simulink model "Kalman_gefiltert"  (R2019b)
settings: Solver=VariableStepAuto  StartTime=0.0  StopTime=750  RelTol=1e-3
undefined symbols (not defined in the file or in its folder): Discrete, Time
libraries: ctrlSharedLib x9

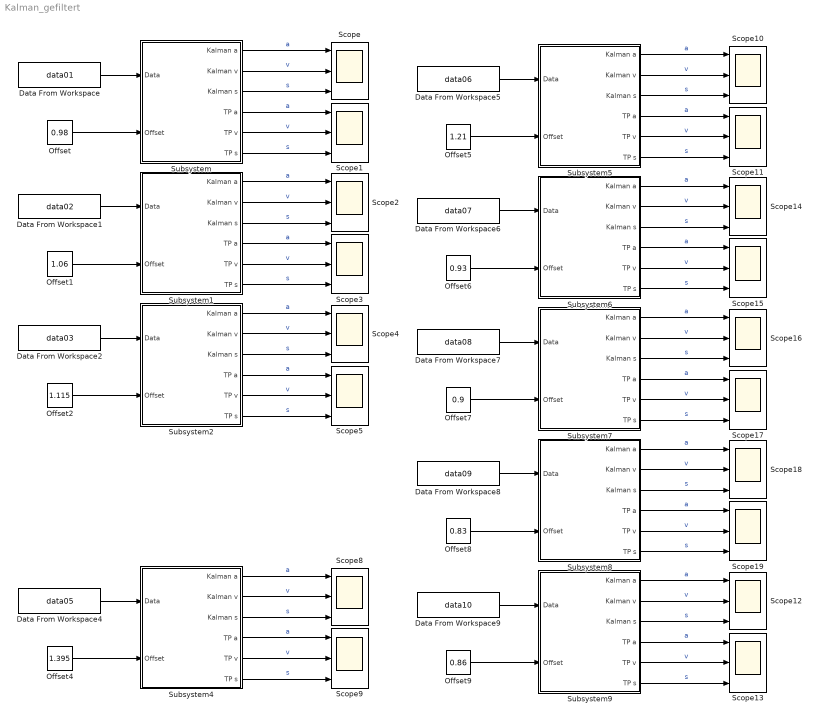
== system Kalman_gefiltert ==
  Data From Workspace : FromWorkspace  VariableName=data01  SampleTime=0
  Data From Workspace1 : FromWorkspace  VariableName=data02  SampleTime=0
  Data From Workspace2 : FromWorkspace  VariableName=data03  SampleTime=0
  Data From Workspace4 : FromWorkspace  VariableName=data05  SampleTime=0
  Data From Workspace5 : FromWorkspace  VariableName=data06  SampleTime=0
  Data From Workspace6 : FromWorkspace  VariableName=data07  SampleTime=0
  Data From Workspace7 : FromWorkspace  VariableName=data08  SampleTime=0
  Data From Workspace8 : FromWorkspace  VariableName=data09  SampleTime=0
  Data From Workspace9 : FromWorkspace  VariableName=data10  SampleTime=0
  Offset : Constant  Value=0.98
  Offset1 : Constant  Value=1.06
  Offset2 : Constant  Value=1.115
  Offset4 : Constant  Value=1.395
  Offset5 : Constant  Value=1.21
  Offset6 : Constant  Value=0.93
  Offset7 : Constant  Value=0.9
  Offset8 : Constant  Value=0.83
  Offset9 : Constant  Value=0.86
  Scope{,1..5,8..19} (18 alike) : Scope  NumInputPorts=3
  Subsystem : Subsystem
  Subsystem1 : Subsystem
  Subsystem2 : Subsystem
  Subsystem4 : Subsystem
  Subsystem5 : Subsystem
  Subsystem6 : Subsystem
  Subsystem7 : Subsystem
  Subsystem8 : Subsystem
  Subsystem9 : Subsystem
  wires:
  Data From Workspace/1 -> Subsystem/1(Data)
  Offset/1 -> Subsystem/2(Offset)
  Subsystem/1(Kalman a) -> Scope/1  "a"
  Subsystem/2(Kalman v) -> Scope/2  "v"
  Subsystem/3(Kalman s) -> Scope/3  "s"
  Subsystem/4(TP a) -> Scope1/1  "a"
  Subsystem/5(TP v) -> Scope1/2  "v"
  Subsystem/6(TP s) -> Scope1/3  "s"
  Subsystem1/6(TP s) -> Scope3/3  "s"
  Subsystem1/5(TP v) -> Scope3/2  "v"
  Subsystem1/3(Kalman s) -> Scope2/3  "s"
  Offset1/1 -> Subsystem1/2(Offset)
  Subsystem1/2(Kalman v) -> Scope2/2  "v"
  Subsystem1/4(TP a) -> Scope3/1  "a"
  Subsystem1/1(Kalman a) -> Scope2/1  "a"
  Data From Workspace2/1 -> Subsystem2/1(Data)
  Subsystem2/6(TP s) -> Scope5/3  "s"
  Subsystem2/5(TP v) -> Scope5/2  "v"
  Subsystem2/3(Kalman s) -> Scope4/3  "s"
  Offset2/1 -> Subsystem2/2(Offset)
  Subsystem2/2(Kalman v) -> Scope4/2  "v"
  Subsystem2/4(TP a) -> Scope5/1  "a"
  Subsystem2/1(Kalman a) -> Scope4/1  "a"
  Subsystem5/2(Kalman v) -> Scope10/2  "v"
  Subsystem5/1(Kalman a) -> Scope10/1  "a"
  Offset5/1 -> Subsystem5/2(Offset)
  Subsystem5/4(TP a) -> Scope11/1  "a"
  Subsystem5/5(TP v) -> Scope11/2  "v"
  Subsystem5/3(Kalman s) -> Scope10/3  "s"
  Data From Workspace5/1 -> Subsystem5/1(Data)
  Subsystem4/1(Kalman a) -> Scope8/1  "a"
  Offset4/1 -> Subsystem4/2(Offset)
  Subsystem4/3(Kalman s) -> Scope8/3  "s"
  Subsystem4/2(Kalman v) -> Scope8/2  "v"
  Subsystem4/5(TP v) -> Scope9/2  "v"
  Data From Workspace4/1 -> Subsystem4/1(Data)
  Subsystem4/4(TP a) -> Scope9/1  "a"
  Subsystem4/6(TP s) -> Scope9/3  "s"
  Subsystem5/6(TP s) -> Scope11/3  "s"
  Subsystem7/1(Kalman a) -> Scope16/1  "a"
  Subsystem9/6(TP s) -> Scope13/3  "s"
  Subsystem8/6(TP s) -> Scope19/3  "s"
  Data From Workspace8/1 -> Subsystem8/1(Data)
  Subsystem8/1(Kalman a) -> Scope18/1  "a"
  Subsystem8/4(TP a) -> Scope19/1  "a"
  Subsystem8/5(TP v) -> Scope19/2  "v"
  Subsystem7/3(Kalman s) -> Scope16/3  "s"
  Offset9/1 -> Subsystem9/2(Offset)
  Subsystem9/4(TP a) -> Scope13/1  "a"
  Data From Workspace9/1 -> Subsystem9/1(Data)
  Subsystem9/3(Kalman s) -> Scope12/3  "s"
  Subsystem8/2(Kalman v) -> Scope18/2  "v"
  Subsystem9/5(TP v) -> Scope13/2  "v"
  Subsystem7/4(TP a) -> Scope17/1  "a"
  Data From Workspace7/1 -> Subsystem7/1(Data)
  Subsystem7/2(Kalman v) -> Scope16/2  "v"
  Subsystem8/3(Kalman s) -> Scope18/3  "s"
  Offset7/1 -> Subsystem7/2(Offset)
  Subsystem7/6(TP s) -> Scope17/3  "s"
  Subsystem6/1(Kalman a) -> Scope14/1  "a"
  Offset6/1 -> Subsystem6/2(Offset)
  Subsystem9/1(Kalman a) -> Scope12/1  "a"
  Offset8/1 -> Subsystem8/2(Offset)
  Subsystem6/4(TP a) -> Scope15/1  "a"
  Subsystem6/5(TP v) -> Scope15/2  "v"
  Subsystem6/2(Kalman v) -> Scope14/2  "v"
  Subsystem7/5(TP v) -> Scope17/2  "v"
  Data From Workspace6/1 -> Subsystem6/1(Data)
  Subsystem6/6(TP s) -> Scope15/3  "s"
  Subsystem6/3(Kalman s) -> Scope14/3  "s"
  Subsystem9/2(Kalman v) -> Scope12/2  "v"
  Data From Workspace1/1 -> Subsystem1/1(Data)

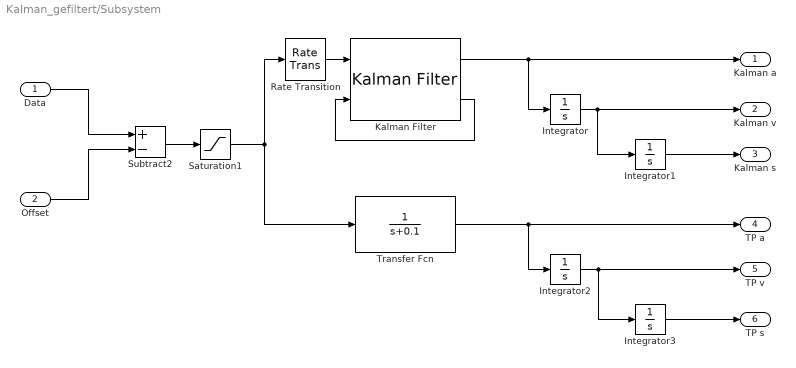
== system Kalman_gefiltert/Subsystem ==
  Data : Inport
  Offset : Inport  Port=2
  Integrator{,1..3} (4 alike) : Integrator
  Kalman Filter : ctrlSharedLib/Kalman Filter  TimeDomain=Discrete-Time  UseCurrentEstimator=on  ModelSource=LTI State-Space Variable  ModelSourceVariable=ss(0.95,1,1,0,1)  A=0.95  B=1  C=1  D=0  NumberOfStates=1  NumberOfInputs=1  NumberOfOutputs=1  InitialEstimateSource=Dialog  X0=0  P0=10  UseK=off  UseGH=off  NumberOfProcessNoiseInputs=1  G=1  TimeInvariantG=on  H=0  TimeInvariantH=on  Q=0.05  TimeInvariantQ=on  R=1  TimeInvariantR=on  N=0  TimeInvariantN=on  AddInputPort=on  AddEnablePort=off  OutputEstimatedY=on  OutputP=off  Ts=-1
  Rate Transition : RateTransition
  Saturation1 : Saturate  UpperLimit=inf  LowerLimit=0
  Subtract2 : Sum  Inputs=+-
  Transfer Fcn : TransferFcn  Denominator=[1 0.1]
  Kalman a : Outport
  Kalman v : Outport  Port=2
  Kalman s : Outport  Port=3
  TP a : Outport  Port=4
  TP v : Outport  Port=5
  TP s : Outport  Port=6
  wires:
  Integrator2/1 -> TP v/1, Integrator3/1
  Integrator3/1 -> TP s/1
  Kalman Filter/2 -> Kalman Filter/2
  Data/1 -> Subtract2/1
  Offset/1 -> Subtract2/2
  Integrator/1 -> Kalman v/1, Integrator1/1
  Transfer Fcn/1 -> TP a/1, Integrator2/1
  Subtract2/1 -> Saturation1/1
  Kalman Filter/1 -> Kalman a/1, Integrator/1
  Integrator1/1 -> Kalman s/1
  Saturation1/1 -> Transfer Fcn/1, Rate Transition/1
  Rate Transition/1 -> Kalman Filter/1

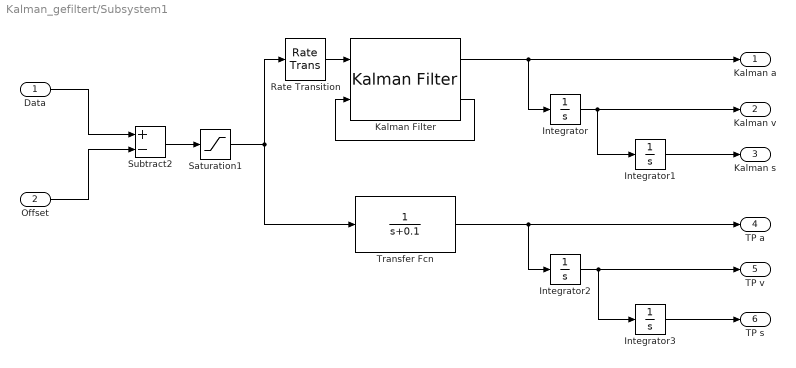
== system Kalman_gefiltert/Subsystem1 ==
  Data : Inport
  Offset : Inport  Port=2
  Integrator{,1..3} (4 alike) : Integrator
  Kalman Filter : ctrlSharedLib/Kalman Filter  TimeDomain=Discrete-Time  UseCurrentEstimator=on  ModelSource=LTI State-Space Variable  ModelSourceVariable=ss(0.95,1,1,0,1)  A=0.95  B=1  C=1  D=0  NumberOfStates=1  NumberOfInputs=1  NumberOfOutputs=1  InitialEstimateSource=Dialog  X0=0  P0=10  UseK=off  UseGH=off  NumberOfProcessNoiseInputs=1  G=1  TimeInvariantG=on  H=0  TimeInvariantH=on  Q=0.05  TimeInvariantQ=on  R=1  TimeInvariantR=on  N=0  TimeInvariantN=on  AddInputPort=on  AddEnablePort=off  OutputEstimatedY=on  OutputP=off  Ts=-1
  Rate Transition : RateTransition
  Saturation1 : Saturate  UpperLimit=inf  LowerLimit=0
  Subtract2 : Sum  Inputs=+-
  Transfer Fcn : TransferFcn  Denominator=[1 0.1]
  Kalman a : Outport
  Kalman v : Outport  Port=2
  Kalman s : Outport  Port=3
  TP a : Outport  Port=4
  TP v : Outport  Port=5
  TP s : Outport  Port=6
  wires:
  Integrator2/1 -> TP v/1, Integrator3/1
  Integrator3/1 -> TP s/1
  Kalman Filter/2 -> Kalman Filter/2
  Data/1 -> Subtract2/1
  Offset/1 -> Subtract2/2
  Integrator/1 -> Kalman v/1, Integrator1/1
  Transfer Fcn/1 -> TP a/1, Integrator2/1
  Subtract2/1 -> Saturation1/1
  Kalman Filter/1 -> Kalman a/1, Integrator/1
  Integrator1/1 -> Kalman s/1
  Saturation1/1 -> Transfer Fcn/1, Rate Transition/1
  Rate Transition/1 -> Kalman Filter/1

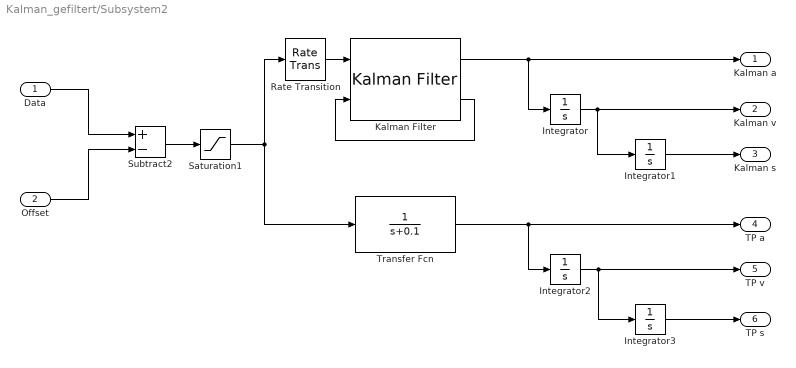
== system Kalman_gefiltert/Subsystem2 ==
  Data : Inport
  Offset : Inport  Port=2
  Integrator{,1..3} (4 alike) : Integrator
  Kalman Filter : ctrlSharedLib/Kalman Filter  TimeDomain=Discrete-Time  UseCurrentEstimator=on  ModelSource=LTI State-Space Variable  ModelSourceVariable=ss(0.95,1,1,0,1)  A=0.95  B=1  C=1  D=0  NumberOfStates=1  NumberOfInputs=1  NumberOfOutputs=1  InitialEstimateSource=Dialog  X0=0  P0=10  UseK=off  UseGH=off  NumberOfProcessNoiseInputs=1  G=1  TimeInvariantG=on  H=0  TimeInvariantH=on  Q=0.05  TimeInvariantQ=on  R=1  TimeInvariantR=on  N=0  TimeInvariantN=on  AddInputPort=on  AddEnablePort=off  OutputEstimatedY=on  OutputP=off  Ts=-1
  Rate Transition : RateTransition
  Saturation1 : Saturate  UpperLimit=inf  LowerLimit=0
  Subtract2 : Sum  Inputs=+-
  Transfer Fcn : TransferFcn  Denominator=[1 0.1]
  Kalman a : Outport
  Kalman v : Outport  Port=2
  Kalman s : Outport  Port=3
  TP a : Outport  Port=4
  TP v : Outport  Port=5
  TP s : Outport  Port=6
  wires:
  Integrator2/1 -> TP v/1, Integrator3/1
  Integrator3/1 -> TP s/1
  Kalman Filter/2 -> Kalman Filter/2
  Data/1 -> Subtract2/1
  Offset/1 -> Subtract2/2
  Integrator/1 -> Kalman v/1, Integrator1/1
  Transfer Fcn/1 -> TP a/1, Integrator2/1
  Subtract2/1 -> Saturation1/1
  Kalman Filter/1 -> Kalman a/1, Integrator/1
  Integrator1/1 -> Kalman s/1
  Saturation1/1 -> Transfer Fcn/1, Rate Transition/1
  Rate Transition/1 -> Kalman Filter/1

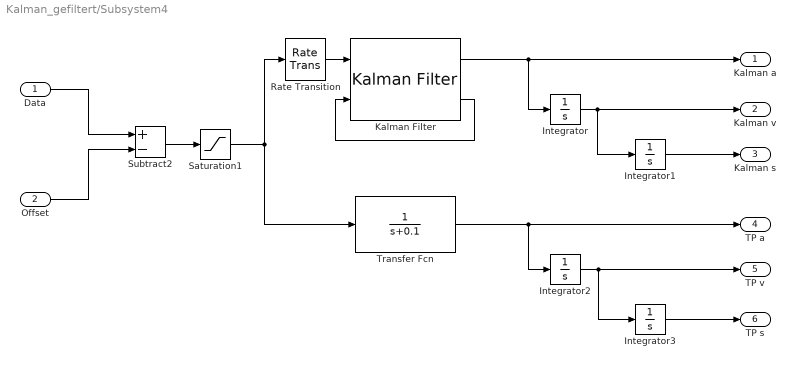
== system Kalman_gefiltert/Subsystem4 ==
  Data : Inport
  Offset : Inport  Port=2
  Integrator{,1..3} (4 alike) : Integrator
  Kalman Filter : ctrlSharedLib/Kalman Filter  TimeDomain=Discrete-Time  UseCurrentEstimator=on  ModelSource=LTI State-Space Variable  ModelSourceVariable=ss(0.95,1,1,0,1)  A=0.95  B=1  C=1  D=0  NumberOfStates=1  NumberOfInputs=1  NumberOfOutputs=1  InitialEstimateSource=Dialog  X0=0  P0=10  UseK=off  UseGH=off  NumberOfProcessNoiseInputs=1  G=1  TimeInvariantG=on  H=0  TimeInvariantH=on  Q=0.05  TimeInvariantQ=on  R=1  TimeInvariantR=on  N=0  TimeInvariantN=on  AddInputPort=on  AddEnablePort=off  OutputEstimatedY=on  OutputP=off  Ts=-1
  Rate Transition : RateTransition
  Saturation1 : Saturate  UpperLimit=inf  LowerLimit=0
  Subtract2 : Sum  Inputs=+-
  Transfer Fcn : TransferFcn  Denominator=[1 0.1]
  Kalman a : Outport
  Kalman v : Outport  Port=2
  Kalman s : Outport  Port=3
  TP a : Outport  Port=4
  TP v : Outport  Port=5
  TP s : Outport  Port=6
  wires:
  Integrator2/1 -> TP v/1, Integrator3/1
  Integrator3/1 -> TP s/1
  Kalman Filter/2 -> Kalman Filter/2
  Data/1 -> Subtract2/1
  Offset/1 -> Subtract2/2
  Integrator/1 -> Kalman v/1, Integrator1/1
  Transfer Fcn/1 -> TP a/1, Integrator2/1
  Subtract2/1 -> Saturation1/1
  Kalman Filter/1 -> Kalman a/1, Integrator/1
  Integrator1/1 -> Kalman s/1
  Saturation1/1 -> Transfer Fcn/1, Rate Transition/1
  Rate Transition/1 -> Kalman Filter/1

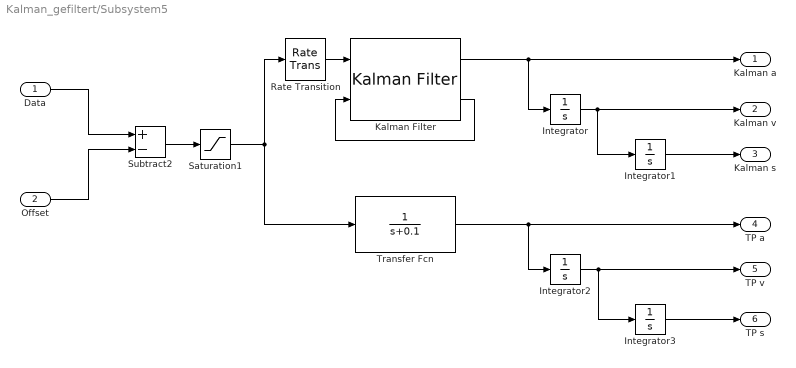
== system Kalman_gefiltert/Subsystem5 ==
  Data : Inport
  Offset : Inport  Port=2
  Integrator{,1..3} (4 alike) : Integrator
  Kalman Filter : ctrlSharedLib/Kalman Filter  TimeDomain=Discrete-Time  UseCurrentEstimator=on  ModelSource=LTI State-Space Variable  ModelSourceVariable=ss(0.95,1,1,0,1)  A=0.95  B=1  C=1  D=0  NumberOfStates=1  NumberOfInputs=1  NumberOfOutputs=1  InitialEstimateSource=Dialog  X0=0  P0=10  UseK=off  UseGH=off  NumberOfProcessNoiseInputs=1  G=1  TimeInvariantG=on  H=0  TimeInvariantH=on  Q=0.05  TimeInvariantQ=on  R=1  TimeInvariantR=on  N=0  TimeInvariantN=on  AddInputPort=on  AddEnablePort=off  OutputEstimatedY=on  OutputP=off  Ts=-1
  Rate Transition : RateTransition
  Saturation1 : Saturate  UpperLimit=inf  LowerLimit=0
  Subtract2 : Sum  Inputs=+-
  Transfer Fcn : TransferFcn  Denominator=[1 0.1]
  Kalman a : Outport
  Kalman v : Outport  Port=2
  Kalman s : Outport  Port=3
  TP a : Outport  Port=4
  TP v : Outport  Port=5
  TP s : Outport  Port=6
  wires:
  Integrator2/1 -> TP v/1, Integrator3/1
  Integrator3/1 -> TP s/1
  Kalman Filter/2 -> Kalman Filter/2
  Data/1 -> Subtract2/1
  Offset/1 -> Subtract2/2
  Integrator/1 -> Kalman v/1, Integrator1/1
  Transfer Fcn/1 -> TP a/1, Integrator2/1
  Subtract2/1 -> Saturation1/1
  Kalman Filter/1 -> Kalman a/1, Integrator/1
  Integrator1/1 -> Kalman s/1
  Saturation1/1 -> Transfer Fcn/1, Rate Transition/1
  Rate Transition/1 -> Kalman Filter/1

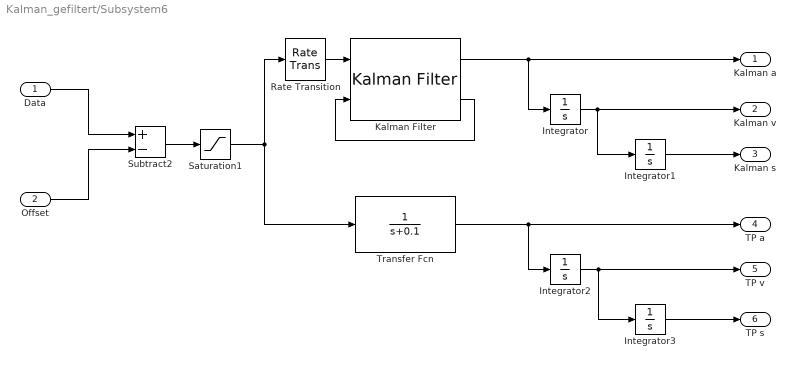
== system Kalman_gefiltert/Subsystem6 ==
  Data : Inport
  Offset : Inport  Port=2
  Integrator{,1..3} (4 alike) : Integrator
  Kalman Filter : ctrlSharedLib/Kalman Filter  TimeDomain=Discrete-Time  UseCurrentEstimator=on  ModelSource=LTI State-Space Variable  ModelSourceVariable=ss(0.95,1,1,0,1)  A=0.95  B=1  C=1  D=0  NumberOfStates=1  NumberOfInputs=1  NumberOfOutputs=1  InitialEstimateSource=Dialog  X0=0  P0=10  UseK=off  UseGH=off  NumberOfProcessNoiseInputs=1  G=1  TimeInvariantG=on  H=0  TimeInvariantH=on  Q=0.05  TimeInvariantQ=on  R=1  TimeInvariantR=on  N=0  TimeInvariantN=on  AddInputPort=on  AddEnablePort=off  OutputEstimatedY=on  OutputP=off  Ts=-1
  Rate Transition : RateTransition
  Saturation1 : Saturate  UpperLimit=inf  LowerLimit=0
  Subtract2 : Sum  Inputs=+-
  Transfer Fcn : TransferFcn  Denominator=[1 0.1]
  Kalman a : Outport
  Kalman v : Outport  Port=2
  Kalman s : Outport  Port=3
  TP a : Outport  Port=4
  TP v : Outport  Port=5
  TP s : Outport  Port=6
  wires:
  Integrator2/1 -> TP v/1, Integrator3/1
  Integrator3/1 -> TP s/1
  Kalman Filter/2 -> Kalman Filter/2
  Data/1 -> Subtract2/1
  Offset/1 -> Subtract2/2
  Integrator/1 -> Kalman v/1, Integrator1/1
  Transfer Fcn/1 -> TP a/1, Integrator2/1
  Subtract2/1 -> Saturation1/1
  Kalman Filter/1 -> Kalman a/1, Integrator/1
  Integrator1/1 -> Kalman s/1
  Saturation1/1 -> Transfer Fcn/1, Rate Transition/1
  Rate Transition/1 -> Kalman Filter/1

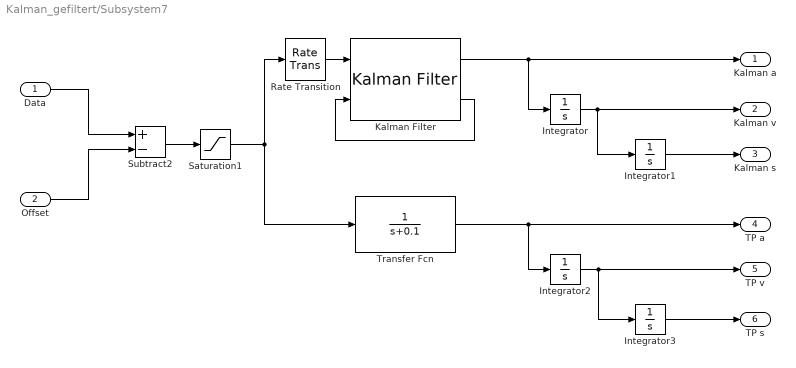
== system Kalman_gefiltert/Subsystem7 ==
  Data : Inport
  Offset : Inport  Port=2
  Integrator{,1..3} (4 alike) : Integrator
  Kalman Filter : ctrlSharedLib/Kalman Filter  TimeDomain=Discrete-Time  UseCurrentEstimator=on  ModelSource=LTI State-Space Variable  ModelSourceVariable=ss(0.95,1,1,0,1)  A=0.95  B=1  C=1  D=0  NumberOfStates=1  NumberOfInputs=1  NumberOfOutputs=1  InitialEstimateSource=Dialog  X0=0  P0=10  UseK=off  UseGH=off  NumberOfProcessNoiseInputs=1  G=1  TimeInvariantG=on  H=0  TimeInvariantH=on  Q=0.05  TimeInvariantQ=on  R=1  TimeInvariantR=on  N=0  TimeInvariantN=on  AddInputPort=on  AddEnablePort=off  OutputEstimatedY=on  OutputP=off  Ts=-1
  Rate Transition : RateTransition
  Saturation1 : Saturate  UpperLimit=inf  LowerLimit=0
  Subtract2 : Sum  Inputs=+-
  Transfer Fcn : TransferFcn  Denominator=[1 0.1]
  Kalman a : Outport
  Kalman v : Outport  Port=2
  Kalman s : Outport  Port=3
  TP a : Outport  Port=4
  TP v : Outport  Port=5
  TP s : Outport  Port=6
  wires:
  Integrator2/1 -> TP v/1, Integrator3/1
  Integrator3/1 -> TP s/1
  Kalman Filter/2 -> Kalman Filter/2
  Data/1 -> Subtract2/1
  Offset/1 -> Subtract2/2
  Integrator/1 -> Kalman v/1, Integrator1/1
  Transfer Fcn/1 -> TP a/1, Integrator2/1
  Subtract2/1 -> Saturation1/1
  Kalman Filter/1 -> Kalman a/1, Integrator/1
  Integrator1/1 -> Kalman s/1
  Saturation1/1 -> Transfer Fcn/1, Rate Transition/1
  Rate Transition/1 -> Kalman Filter/1

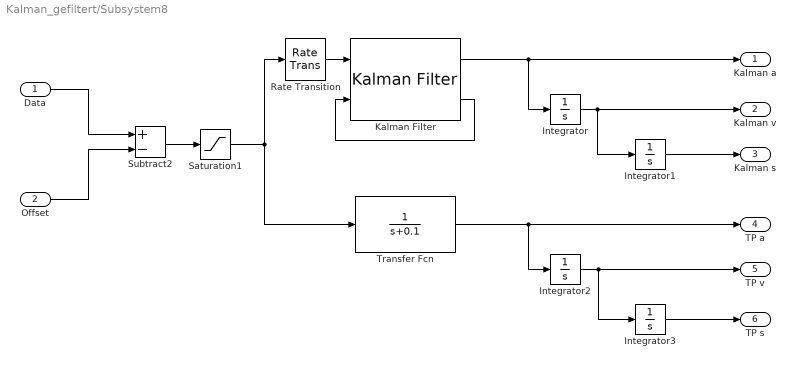
== system Kalman_gefiltert/Subsystem8 ==
  Data : Inport
  Offset : Inport  Port=2
  Integrator{,1..3} (4 alike) : Integrator
  Kalman Filter : ctrlSharedLib/Kalman Filter  TimeDomain=Discrete-Time  UseCurrentEstimator=on  ModelSource=LTI State-Space Variable  ModelSourceVariable=ss(0.95,1,1,0,1)  A=0.95  B=1  C=1  D=0  NumberOfStates=1  NumberOfInputs=1  NumberOfOutputs=1  InitialEstimateSource=Dialog  X0=0  P0=10  UseK=off  UseGH=off  NumberOfProcessNoiseInputs=1  G=1  TimeInvariantG=on  H=0  TimeInvariantH=on  Q=0.05  TimeInvariantQ=on  R=1  TimeInvariantR=on  N=0  TimeInvariantN=on  AddInputPort=on  AddEnablePort=off  OutputEstimatedY=on  OutputP=off  Ts=-1
  Rate Transition : RateTransition
  Saturation1 : Saturate  UpperLimit=inf  LowerLimit=0
  Subtract2 : Sum  Inputs=+-
  Transfer Fcn : TransferFcn  Denominator=[1 0.1]
  Kalman a : Outport
  Kalman v : Outport  Port=2
  Kalman s : Outport  Port=3
  TP a : Outport  Port=4
  TP v : Outport  Port=5
  TP s : Outport  Port=6
  wires:
  Integrator2/1 -> TP v/1, Integrator3/1
  Integrator3/1 -> TP s/1
  Kalman Filter/2 -> Kalman Filter/2
  Data/1 -> Subtract2/1
  Offset/1 -> Subtract2/2
  Integrator/1 -> Kalman v/1, Integrator1/1
  Transfer Fcn/1 -> TP a/1, Integrator2/1
  Subtract2/1 -> Saturation1/1
  Kalman Filter/1 -> Kalman a/1, Integrator/1
  Integrator1/1 -> Kalman s/1
  Saturation1/1 -> Transfer Fcn/1, Rate Transition/1
  Rate Transition/1 -> Kalman Filter/1

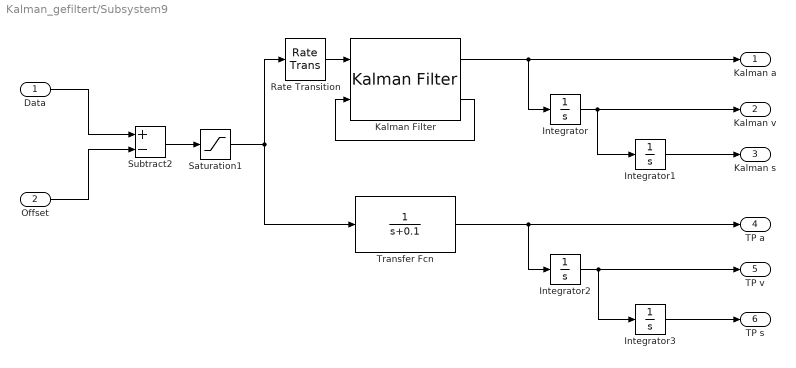
== system Kalman_gefiltert/Subsystem9 ==
  Data : Inport
  Offset : Inport  Port=2
  Integrator{,1..3} (4 alike) : Integrator
  Kalman Filter : ctrlSharedLib/Kalman Filter  TimeDomain=Discrete-Time  UseCurrentEstimator=on  ModelSource=LTI State-Space Variable  ModelSourceVariable=ss(0.95,1,1,0,1)  A=0.95  B=1  C=1  D=0  NumberOfStates=1  NumberOfInputs=1  NumberOfOutputs=1  InitialEstimateSource=Dialog  X0=0  P0=10  UseK=off  UseGH=off  NumberOfProcessNoiseInputs=1  G=1  TimeInvariantG=on  H=0  TimeInvariantH=on  Q=0.05  TimeInvariantQ=on  R=1  TimeInvariantR=on  N=0  TimeInvariantN=on  AddInputPort=on  AddEnablePort=off  OutputEstimatedY=on  OutputP=off  Ts=-1
  Rate Transition : RateTransition
  Saturation1 : Saturate  UpperLimit=inf  LowerLimit=0
  Subtract2 : Sum  Inputs=+-
  Transfer Fcn : TransferFcn  Denominator=[1 0.1]
  Kalman a : Outport
  Kalman v : Outport  Port=2
  Kalman s : Outport  Port=3
  TP a : Outport  Port=4
  TP v : Outport  Port=5
  TP s : Outport  Port=6
  wires:
  Integrator2/1 -> TP v/1, Integrator3/1
  Integrator3/1 -> TP s/1
  Kalman Filter/2 -> Kalman Filter/2
  Data/1 -> Subtract2/1
  Offset/1 -> Subtract2/2
  Integrator/1 -> Kalman v/1, Integrator1/1
  Transfer Fcn/1 -> TP a/1, Integrator2/1
  Subtract2/1 -> Saturation1/1
  Kalman Filter/1 -> Kalman a/1, Integrator/1
  Integrator1/1 -> Kalman s/1
  Saturation1/1 -> Transfer Fcn/1, Rate Transition/1
  Rate Transition/1 -> Kalman Filter/1
